simulink model "QuarkControl"  (R2018a)
settings: Solver=FixedStepAuto  StartTime=0.0  StopTime=20  FixedStep=0.004  RelTol=1e-3
InitFcn:
  | seed1 = rand()*1000000;
  | seed2 = rand()*1000000;
  | seed3 = rand()*1000000;
libraries: quarc_library x1
settings Model: SimulationMode=external  ExtModeTrigDuration=5000  Creator=RSamra  LastModifiedBy=李玉玲
settings SolverCC: PositivePriorityOrder=on  AutoInsertRateTranBlk=on
settings DataIOCC: LimitDataPoints=on  SaveFormat=Array  SignalLoggingSaveFormat=ModelDataLogs  ReturnWorkspaceOutputs=on
settings OptimizationCC: ExpressionDepthLimit=2147483647  InitFltsAndDblsToZero=on  LifeSpan=inf
settings DebuggingCC: UnderspecifiedInitializationDetection=Classic  MergeDetectMultiDrivingBlocksExec=none  SolverPrmCheckMsg=warning  FcnCallInpInsideContextMsg=warning  StateNameClashWarn=warning  SFUnexpectedBacktrackingDiag=warning  SFNoUnconditionalDefaultTransitionDiag=warning  SFExecutionAtInitializationDiag=none
settings HardwareCC: ProdBitPerPointer=32  ProdBitPerSizeT=32  ProdBitPerPtrDiffT=32  ProdLargestAtomicFloat=None  ProdIntDivRoundTo=Undefined  ProdEndianess=Unspecified  ProdWordSize=32  ProdHWDeviceType=32-bit Generic
settings ModelReferenceCC: PropagateSignalLabelsOutOfModel=off
settings SFSimCC: SimParseCustomCode=off
settings RTWCC: SystemTargetFile=quarc_win64.tlc  TemplateMakefile=quarc_default_tmf  Description=QUARC Win64 Target
settings CodeAppCC: StateflowObjectComments=on
settings STFCustomTargetCC: TargetPreCompLibLocation=C:\PROGRA~3\QUARC\lib\2018a\win64\release  ConcurrentExecutionCompliant=on  CombineOutputUpdateFcns=on  CPPClassGenCompliant=on  GRTInterface=off  SystemTargetFile=quarc_win64.tlc
settings GRTTargetCC: TargetPreCompLibLocation=C:\PROGRA~3\QUARC\lib\2018a\win64\release  TargetLangStandard=C89/C90 (ANSI)  ParMdlRefBuildCompliant=off  CompOptLevelCompliant=off  MatFileLogging=off  UseToolchainInfoCompliant=off  ExtMode=on  ExtModeMexFile=quarc_comm
settings ConfigComp: CovMetricSettings=dw  CovSaveCumulativeToWorkspaceVar=on  CovSaveSingleToWorkspaceVar=on  CovExternalEMLEnable=off

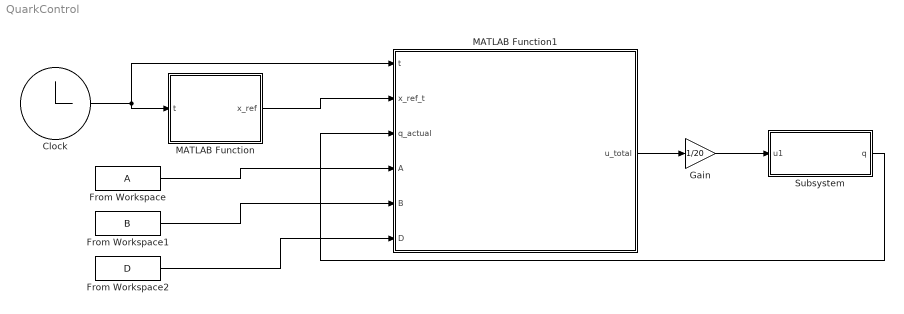
== system QuarkControl ==
  Clock : Clock
      settings: Decimation=99999999
  From Workspace : FromWorkspace  VariableName=A  SampleTime=0
  From Workspace1 : FromWorkspace  VariableName=B  SampleTime=0
  From Workspace2 : FromWorkspace  VariableName=D  SampleTime=0
  Gain : Gain  Gain=1/20
  MATLAB Function : MATLAB Function  TreatAsAtomicUnit=on
  MATLAB Function1 : MATLAB Function  TreatAsAtomicUnit=on
  Subsystem : Subsystem
  wires:
  Clock/1 -> MATLAB Function1/1(t), MATLAB Function/1(t)
  MATLAB Function/1(x_ref) -> MATLAB Function1/2(x_ref_t)
  MATLAB Function1/1(u_total) -> Gain/1
  Subsystem/1(q) -> MATLAB Function1/3(q_actual)
  From Workspace/1 -> MATLAB Function1/4(A)
  From Workspace1/1 -> MATLAB Function1/5(B)
  From Workspace2/1 -> MATLAB Function1/6(D)
  Gain/1 -> Subsystem/1(u1)

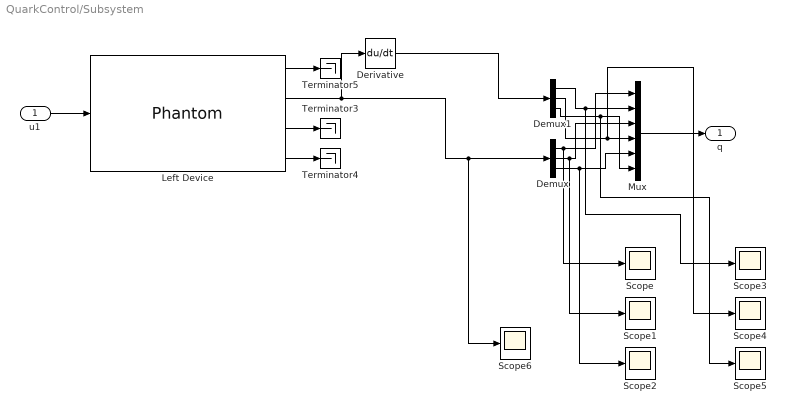
== system QuarkControl/Subsystem ==
  u1 : Inport  PortDimensions=[3 1]
  Demux : Demux  Outputs=3
  Demux1 : Demux  Outputs=3
  Derivative : Derivative
  Left Device : quarc_library/Devices/Third-Party/SensAble/Phantom/Phantom  device_name=Default Device  output_type=Joint and Gimbal Angles  input_type=Joint space  velocity_limit_option=off  velocity_limit=1200  is_7dof=off  sample_time=0.004
      settings: AttributesFormatString=(%<device_name>)  SourceProductName=QUARC Targets
  Mux : Mux  Inputs=6
  Scope{,1..6} (7 alike) : Scope
  Terminator3 : Terminator
  Terminator4 : Terminator
  Terminator5 : Terminator
  q : Outport  PortDimensions=[6 1]
  wires:
  u1/1 -> Left Device/1
  Left Device/2 -> Scope6/1, Demux/1, Derivative/1
  Derivative/1 -> Demux1/1
  Left Device/3 -> Terminator3/1
  Left Device/4 -> Terminator4/1
  Left Device/1 -> Terminator5/1
  Demux/1 -> Scope/1, Mux/1
  Demux/2 -> Scope1/1, Mux/3
  Demux/3 -> Scope2/1, Mux/5
  Demux1/1 -> Scope3/1, Mux/2
  Demux1/2 -> Scope4/1, Mux/4
  Demux1/3 -> Scope5/1, Mux/6
  Mux/1 -> q/1

== matlab function QuarkControl/MATLAB Function1 ==
  data: t input; u_total output; x_ref_t input; q_actual input; A input; B input; D input
function u_total = koopman_lqr_controller(t, x_ref_t, q_actual, A, B, D)
% 描述:
% Koopman LQR 轨迹跟踪控制器 (前馈 + 反馈)
%
% 输入:
%   t:        当前时间 (来自 Clock)
%   x_ref_t:  当前时刻的期望轨迹 [6x1] (来自模块1)
%   q_actual: 当前时刻的实际状态 [6x1] (来自系统反馈)
%   A:        Koopman 状态矩阵 [z_dim x z_dim] (来自工作区)
%   B:        Koopman 控制矩阵 [z_dim x p] (来自工作区)
%   D:        特征选择矩阵 [N x P] (来自工作区)
%
% 输出:
%   u_total:  计算得到的控制力矩 [p x 1]

% --- 1. 定义系统维度 ---
n = size(q_actual, 1); % n=6
p = size(B, 2);      % p=3
N = size(D, 1);      % N
z_dim = n + N;

% --- 2. 时间检查 (按要求 t < 10 时输出 0) ---
if t < 10.0
    u_total = zeros(p, 1);
    return;
end

% --- 3. 定义控制器内部参数 (使用 persistent 提高效率) ---
% persistent 变量只在第一次运行时计算一次，
% 避免在每个Simulink步长都重新计算LQR增益。

persistent K_lqr B_pinv is_initialized;

if isempty(is_initialized)
    % 1. 定义C矩阵 (如您所要求)
    % C_model = [eye(n), zeros(n, N)]; % (C矩阵在控制器中并未使用)
    
    % 2. 定义LQR惩罚矩阵 Q 和 R
    Q = zeros(z_dim, z_dim);
    % [q1, dq1, q2, dq2, q3, dq3] 的惩罚
    Q_x_diag = [100; 0; 100; 0; 100; 0]; 
    Q(1:n, 1:n) = diag(Q_x_diag);
    
    % R 矩阵 (控制惩罚)
    % 注：R=0 在 dlqr 中是不允许的 (必须是正定)。
    % 使用一个很小的值 (1e-4) 来代替 0。
    R = 0 * eye(p);
    
    % 3. 计算 LQR 增益 (需要 Control System Toolbox)
    K_lqr = dlqr(double(A), double(B), double(Q), double(R));
    
    % 4. 计算 B 的伪逆 (用于前馈)
    B_pinv = pinv(double(B));
    
    is_initialized = true;
end

% --- 4. 仿真步长 (必须与您的Simulink求解器步长一致!) ---
dt = 0.004;

% --- 5. 计算前馈控制 (u_ff) ---
% u_ff(t) = pinv(B) * (z_ref(t+1) - A * z_ref(t))

% 5.1. 抬升当前期望状态 z_ref(t)
z_ref_t = lift_state(x_ref_t, D, n);

% 5.2. 计算下一时刻的期望状态 x_ref(t+1)
t_next = t + dt;
x_ref_t_next = generate_reference_internal(t_next, n);

% 5.3. 抬升下一时刻的期望状态 z_ref(t+1)
z_ref_t_next = lift_state(x_ref_t_next, D, n);

% 5.4. 计算前馈控制
u_ff = B_pinv * (z_ref_t_next - A * z_ref_t);

% --- 6. 计算反馈控制 (u_fb) ---
% u_fb(t) = -K_lqr * (z_actual(t) - z_ref(t))

% 6.1. 抬升当前实际状态 z_actual(t)
z_actual = lift_state(q_actual, D, n);

% 6.2. 计算状态误差
z_error = z_actual - z_ref_t;

% 6.3. 计算反馈控制
u_fb = -K_lqr * z_error;

% --- 7. 计算总控制 ---
u_total = u_ff + u_fb;

end

% =========================================================================
% --- 内部辅助函数 (Internal Helper Functions) ---
% =========================================================================

function z = lift_state(x, D_in, n_in)
    % 辅助函数：将 [n x 1] 的状态 x 抬升到 [z_dim x 1] 的 z
    
    % lift_function 需要 (m x n) 输入, 即 (1 x 6)
    phi_x_row = lift_function(x'); 
    
    % 转换为 (P x 1)
    phi_x_col = phi_x_row';
    
    % z = [x; D*Phi]
    z = [x(1:n_in, 1); D_in * phi_x_col];
end


function x_ref_internal = generate_reference_internal(t_in, n_in)
    % 辅助函数：计算 t_in 时刻的期望轨迹
    % (与模块1的逻辑完全相同)
    
    % --- 1. 定义轨迹参数 ---
    f_pos = 0.1;   % 频率 (Hz)
    omega = 2 * pi * f_pos; % 角频率 (rad/s)
    A1 = 0.3; B1 = 0.0;   % 关节 1
    A2 = 0.2; B2 = 0.865; % 关节 2
    A3 = 0.1; B3 = 1.045; % 关节 3

    % --- 2. 计算位置和速度 ---
    x_ref_internal = zeros(n_in, 1); % 列向量

    pos_ref_1 = A1 * sin(omega * t_in) + B1;
    vel_ref_1 = A1 * omega * cos(omega * t_in);
    pos_ref_2 = A2 * sin(omega * t_in) + B2;
    vel_ref_2 = A2 * omega * cos(omega * t_in);
    pos_ref_3 = A3 * sin(omega * t_in) + B3;
    vel_ref_3 = A3 * omega * cos(omega * t_in);

    % --- 3. 构造输出向量 ---
    x_ref_internal(1) = pos_ref_1;
    x_ref_internal(2) = vel_ref_1;
    x_ref_internal(3) = pos_ref_2;
    x_ref_internal(4) = vel_ref_2;
    x_ref_internal(5) = pos_ref_3;
    x_ref_internal(6) = vel_ref_3;
end


% =========================================================================
% --- 【嵌入的完整基函数库 (已修正)】 ---
% =========================================================================

function y = lift_function(q)
% LIFT_FUNCTION - 635 维扩充版 (a1 - a21)
% 【嵌入版本：用于MATLAB Function模块】

% --- 1. 提取状态 ---
q1=q(:,1);  dq1=q(:,2);
q2=q(:,3);  dq2=q(:,4);
q3=q(:,5);  dq3=q(:,6);

% --- 2. 基础项 (a1) ---
a1 = [q1, dq1, q2, dq2, q3, dq3, ones(size(q1,1),1)];

% --- 3. 三角函数辅助变量 (a2, a3) ---
c1=cos(q1); s1=sin(q1);
c2=cos(q2); s2=sin(q2);
c3=cos(q3); s3=sin(q3);
c2p3 = cos(q2+q3);
s2p3 = sin(q2+q3);
c2m3 = cos(q2-q3);
s2m3 = sin(q2-q3);

a2 = [s1, c1, s2, c2, s3, c3, c2p3, s2p3, c2m3, s2m3, ...
      c2.*s2, c3.*s3, c2p3.*s2p3, s2.*s3, c2.*c3, s2.*s2p3];

c2q2 = cos(2*q2);  s2q2 = sin(2*q2);
c2q3 = cos(2*q3);  s2q3 = sin(2*q3);
c3q2 = cos(3*q2);  s3q2 = sin(3*q2);
c3q3 = cos(3*q3);  s3q3 = sin(3*q3);
c2q2p3 = cos(2*q2+q3);  s2q2p3 = sin(2*q2+q3);
c2q2m3 = cos(2*q2-q3);  s2q2m3 = sin(2*q2-q3);
cq2p2q3 = cos(q2+2*q3);  sq2p2q3 = sin(q2+2*q3);
c2q2p2q3 = cos(2*q2+2*q3); s2q2p2q3 = sin(2*q2+2*q3);

a3 = [c2q2, s2q2, c2q3, s2q3, c3q2, s3q2, c3q3, s3q3, ...
      c2q2p3, s2q2p3, c2q2m3, s2q2m3, cq2p2q3, sq2p2q3, ...
      c2q2p2q3, s2q2p2q3, ...
      cos(q1+q2), sin(q1+q2), cos(q1+q3), sin(q1+q3), ...
      cos(q1+q2+q3), sin(q1+q2+q3), cos(2*(q2+q3)), sin(2*(q2+q3))];

% --- 4. 特征组 a4 - a18 ---
a4 = [c2.^2, c3.^2, c2p3.^2, c2m3.^2, ...
      c2.*c3, c2.*c2p3, c3.*c2p3, c2.*c2m3, ...
      s2.^2, s3.^2, s2p3.^2, s2m3.^2, ...
      s2.*s3, s2.*s2p3, c2q2.*c2q3, ...
      (c2.^2).*(c2p3.^2), c2.^3, c2p3.^3, c3.^3, ...
      c2.*c3.^2, c2p3.*c3.^2, c3.^4];

a5 = [s2q2, s2q2p3, sin(2*q2+2*q3), s2q2m3, sin(2*(q2-q3)), ...
      c2.*s2, c3.*s3, c2p3.*s2p3, c2m3.*s2m3, ...
      c2.*s2p3, s2.*c2p3, c2.*s3, s3.*c2p3, ...
      c2.^2.*c2p3, c2.*c2p3.^2, c2.^2.*c3, c3.^2.*c2p3, ...
      c2.*c3.*c2p3, s2.*s3.*s2p3, ...
      c2q2.*c3, c2.*c2q3, s2q2.*s3, s3.*c2q3, s2q3.*c2, ...
      sin(q2).*cos(q2).*cos(q3), sin(q3).*cos(q2+q3)];

a6 = [dq1.*c2, dq1.*s2, dq1.*c3, dq1.*s3, ...
      dq1.*c2p3, dq1.*s2p3, dq1.*c2m3, dq1.*s2m3, ...
      dq1.*c2.^2, dq1.*c2p3.^2, dq1.*c2.*c2p3, dq1.*c2.*c3, ...
      dq1.*c2.*s2, dq1.*s2q2, dq1.*s2q2p3, dq1.*s3, ...
      dq1.*c2q2, dq1.*c2q3, dq1.*s2q3, dq1.*c3.*s3, ...
      dq1.^2.*c2, dq1.^2.*c2p3, dq1.^2.*s2, dq1.^2.*c3, ...
      dq1.*c3.^2, dq1.*s3.^2, dq1.*c2q3];

a7 = [dq1.*s2, dq2.*s2, dq3.*s2, dq1.*s3, dq2.*s3, dq3.*s3, ...
      dq1.*s2p3, dq2.*s2p3, dq3.*s2p3, dq1.*s2m3, dq2.*s2m3, dq3.*s2m3, ...
      dq1.*c2, dq2.*c2, dq3.*c2, dq1.*c3, dq2.*c3, dq3.*c3, ...
      dq2.*s2q2, dq3.*s2q3, dq2.*c2q2, dq3.*c2q3, ...
      dq1.*s2q2p3, dq2.*s2q2p3, dq3.*s2q3, dq3.*c3q3, ...
      dq2.^2.*s2, dq3.^2.*s3, dq2.^2.*c2, dq3.^2.*c3, ...
      dq1.*dq2.*s2, dq2.*dq3.*s3, dq3.*s3.^2, dq3.*c3.^2, ...
      dq2.*c2.*c3, dq3.*s2.*s3];

a8 = [dq1.*dq2, dq1.*dq3, dq2.*dq3, ...
      s3.*dq1.*dq2, s3.*dq2.*dq3, s3.*dq1.*dq3, ...
      s2.*dq1.*dq2, s2.*dq2.*dq3, s2.*dq1.*dq3, ...
      s2q2.*dq1.*dq2, s2q2.*dq2.*dq3, s2q3.*dq2.*dq3, ...
      c2.*dq1.*dq2, c3.*dq2.*dq3, c2p3.*dq1.*dq3, ...
      dq1.*dq2.*dq3, dq1.*dq2.*s2p3, dq2.*dq3.*c3, ...
      (dq1.*dq2).*c2.^2, (dq2.*dq3).*c3.^2, ...
      (dq1.*dq3).*c2p3, dq1.*dq2.*c2.*c3, ...
      dq2.*dq3.*s2.*s3, (dq1.*dq2.*dq3).*s3, ...
      c3.*dq1.*dq3, s3.*dq1.*dq3.^2, dq2.*dq3.*c3.^2, ...
      dq2.*dq3.*s3.^2, c2q3.*dq2.*dq3];

a9 = [dq1.^2, dq2.^2, dq3.^2, ...
      dq1.^2.*c2, dq1.^2.*s2, dq2.^2.*c3, dq2.^2.*s3, dq3.^2.*c3, dq3.^2.*s3, ...
      s3.*dq3.^2, s3.*dq2.^2, s2.*dq1.^2, ...
      dq1.^3, dq2.^3, dq3.^3, ...
      dq1.^2.*dq2, dq1.^2.*dq3, dq2.^2.*dq3, ...
      sqrt(abs(dq2)), sqrt(abs(dq3)), ...
      sign(dq2).*dq2.^2, sign(dq3).*dq3.^2, ...
      dq2.^2.*c2.^2, dq3.^2.*c3.^2, ...
      dq3.^2.*s3.^2, dq3.^2.*c2q3, dq3.^3.*s3, dq3.^3.*c3, ...
      abs(dq3).^1.5, dq3.^2.*sign(dq3)];

a10 = [q1.^2, q2.^2, q3.^2, q1.*q2, q1.*q3, q2.*q3, ...
       q1.*dq1, q2.*dq2, q3.*dq3, q1.*dq2, q1.*dq3, q2.*dq1, ...
       q2.^3, q3.^3, q2.*q3.^2, q3.^4, ...
       q2.^2.*dq2, q3.^2.*dq3, (q2+q3).*dq2, q3.*dq2, ...
       q3.^2.*dq2, q3.^3.*dq3];

a11 = [c2, c2p3, c3, c2+c2p3, c2-c2p3, ...
       q2.*c2, q3.*c2p3, q3.*c3, ...
       dq2.*c2, dq3.*c2p3, c2.*c2p3, s2.*s2p3, ...
       dq2.*s2, dq3.*s3, (c2+c2p3).^2, ...
       q3.*s3, q3.^2.*c3, dq3.*c3, dq3.*s2p3, ...
       c3.*(c2+c2p3), s3.*(s2+s2p3)];

sd1 = sign(dq1); sd2 = sign(dq2); sd3 = sign(dq3);
a12 = [sd1.*dq1, sd2.*dq2, sd3.*dq3, ...
       sd1.*abs(dq1), sd2.*abs(dq2), sd3.*abs(dq3), ...
       dq1.*abs(dq1), dq2.*abs(dq2), dq3.*abs(dq3), ...
       tanh(10*dq1), tanh(10*dq2), tanh(10*dq3), ...
       dq1./(1+abs(dq1)), dq2./(1+abs(dq2)), dq3./(1+abs(dq3)), ...
       zeros(size(dq2)), zeros(size(dq3)), zeros(size(dq2)), zeros(size(dq3)), ... % 占位符 for max/min
       tanh(5*dq3), tanh(20*dq3), sd3.*abs(dq3).^1.5];

a13 = [dq1.*c2.^2, dq1.*c2p3.^2, dq1.*c2.*c2p3, dq1.*c3.^2, ...
       dq2.*c3, dq2.*c3.^2, dq3.*c3, dq3.*c3.^2, ...
       dq2.*(c2+c2p3), dq3.*(c2+c2p3), ...
       sd1.*dq1.*c2, sd2.*dq2.*c3, sd3.*dq3.*c3, ...
       dq1.*dq2.*c2, dq2.*dq3.*c3, ...
       abs(dq2).*c2, abs(dq3).*c3, dq2.*abs(dq2).*s2, ...
       dq3.*c3.^3, dq3.*s3.^2, abs(dq3).*s3, ...
       dq3.*(c2+c2p3), sd3.*dq3.*s3];

h_denom1 = 1./(1 + 0.1*c2.^2 + 0.1*c2p3.^2);
h_denom2 = 1./(1 + 0.1*c3.^2);
h_denom3 = 1./(1 + 0.05*c3.^2 + 0.05*c2p3.^2);

a14 = [h_denom1, h_denom2, h_denom3, ...
       h_denom1.*dq1, h_denom2.*dq2, h_denom2.*dq3, h_denom3.*dq3, ...
       h_denom1.*c2, h_denom1.*c2p3, h_denom2.*c3, ...
       h_denom1.^2, h_denom2.^2, h_denom3.^2, ...
       h_denom1.*c2.^2, h_denom2.*c3.^2, h_denom3.*c3, ...
       h_denom1.*dq1.^2, h_denom2.*dq2.^2, h_denom1.*dq2, ...
       h_denom2.*dq3.^2, h_denom3.*dq2.*dq3];

a15 = [q2.*dq2.^2, q3.*dq3.^2, q2.*dq3.^2, ...
       dq1.^2.*dq2, dq1.^2.*dq3, dq2.*dq3.^2, dq1.*dq2.^2, ...
       q2.*c2.*dq2, q3.*c3.*dq3, q2.*s2.*dq2, ...
       c2.*dq1.*dq2, c3.*dq2.*dq3, s2.*dq1.^2, ...
       dq1.*dq2.*s2p3, dq1.*dq3.*c2p3, ...
       q2.*dq2.*c2, q3.*dq3.*c3, dq2.^2.*s2q2, ...
       q3.*dq3.^2.*c3, q3.*dq3.^2.*s3, q3.^2.*dq3.*c3, ...
       dq3.^2.*c3, dq1.*dq3.^2];

% 【已修正】dq3./(1DEN+abs(c3)) -> dq3./(1+abs(c3))
a16 = [zeros(size(dq2)), zeros(size(dq3)), ... % 占位符 for max/min
       dq2.*(1+c2.^2), dq3.*(1+c3.^2), ...
       dq2.*(1+0.5*c2p3.^2), dq3.*(1+0.5*c3.^2), ...
       dq1./(1+0.1*abs(dq1)), dq2./(1+0.1*abs(dq2)), dq3./(1+0.1*abs(dq3)), ...
       dq2.*(c2+0.5*c2p3), dq3.*(c3+0.5*c2p3), ...
       dq2.*exp(-0.1*q2.^2), dq3.*exp(-0.1*q3.^2), ...
       dq1.*dq2./(1+abs(dq2)), dq2.*dq3./(1+abs(dq3)), ...
       dq2./(1+abs(sin(q3))), dq3./(1+abs(sin(q3))), ...
       dq1.*c2./(1+abs(c2)), dq2.*c3./(1+abs(c3)), ...
       (dq2+dq3).*c2p3, ...
       dq3./(1+abs(c3)), dq3.*(1+s3.^2), zeros(size(dq3)), ... % 占位符 for max/min
       dq3.*(1+abs(q3)), dq3.*exp(-0.05*abs(q3)), ...
       dq3./(1+0.2*abs(dq3)), dq3.*(c3+c2p3)];

a17 = [dq2 + 0.1*dq3, dq3 + 0.1*dq2, ...
       dq1.*(dq2+dq3), (dq1+dq2).*dq3, ...
       dq2 - 0.1*dq2.^3, dq3 - 0.1*dq3.^3, ...
       dq2.*cos(0.5*q2), dq3.*cos(0.5*q3), ...
       (dq2.*dq3)./(1+abs(dq2)+abs(dq3)), ...
       dq2.*(1-0.1*abs(dq2)), dq3.*(1-0.1*abs(dq3)), ...
       dq1+dq2+dq3, ...
       dq3 + 0.2*dq2, dq3.*(1+0.1*dq2), ...
       dq3.*sin(0.5*q3), dq3 - 0.05*dq3.^3, ...
       (dq3+dq2)./(1+abs(dq3)), dq3./(1+abs(dq2)+abs(dq3))];

a18 = [c3.*s3.*dq3, c3.^2.*s3.*dq3, s3.^2.*dq3, ...
       c2q3.*dq3, s2q3.*dq3.^2, c3q3.*dq3, ...
       dq3.*c3./(1+s3.^2), dq3.*s3./(1+c3.^2), ...
       dq2.*dq3.*c3.*s3, dq1.*dq3.*c3, ...
       q3.*c3.*s3, q3.^2.*dq3.*s3, ...
       dq3.^2.*c3.*s3, (dq2.*dq3).*c3, ...
       abs(dq3).*c3.*s3, dq3.*(c3-s3), ...
       dq3.*(c3+s3).^2, c2p3.*s2p3.*dq3, ...
       dq3.*c3.^2.*s3, q3.*dq3.*(c3+s3)];
   
% --- a19: 耦合项 (30 terms) ---
trig_basis_c = [s3, s2q2, s2q2p2q3, s2q2p3, c2.*s2p3];
vel_basis_c = [dq1.^2, dq2.^2, dq3.^2, dq1.*dq2, dq1.*dq3, dq2.*dq3];

a19_list = [];
for i = 1:size(trig_basis_c, 2)
    for j = 1:size(vel_basis_c, 2)
        a19_list = [a19_list, trig_basis_c(:, i) .* vel_basis_c(:, j)];
    end
end
a19 = a19_list;

% --- a20: 高阶多项式 (100 terms) ---
a20_g1 = [q2.^4, q3.^4, dq1.^4, dq2.^4, dq3.^4]; % 5
a20_g2 = [q2.^5, q3.^5, dq1.^5, dq2.^5, dq3.^5]; % 5
a20_g3 = [q2.^3.*dq1, q2.^3.*dq2, q2.^3.*dq3, q3.^3.*dq1, q3.^3.*dq2, q3.^3.*dq3]; % 6
a20_g4 = [q2.*dq1.^3, q2.*dq2.^3, q2.*dq3.^3, q3.*dq1.^3, q3.*dq2.^3, q3.*dq3.^3]; % 6
a20_g5 = [q2.^2.*dq1.^2, q2.^2.*dq2.^2, q2.^2.*dq3.^2, q3.^2.*dq1.^2, q3.^2.*dq2.^2, q3.^2.*dq3.^2]; % 6
a20_g6 = [dq1.^3.*dq2, dq1.^3.*dq3, dq2.^3.*dq1, dq2.^3.*dq3, dq3.^3.*dq1, dq3.^3.*dq2, ...
          dq1.^2.*dq2.^2, dq1.^2.*dq3.^2, dq2.^2.*dq3.^2, dq1.*dq2.*dq3.^2]; % 10
a20_g7 = [dq1.^4.*dq2, dq1.^4.*dq3, dq2.^4.*dq1, dq2.^4.*dq3, dq3.^4.*dq1, dq3.^4.*dq2, ...
          dq1.^3.*dq2.^2, dq1.^2.*dq2.^3, dq1.^3.*dq3.^2, dq1.^2.*dq3.^3, dq2.^3.*dq3.^2, dq2.^2.*dq3.^3]; % 12
a20_g8 = [q2.^4, q3.^4, q2.^3.*q3, q2.^2.*q3.^2, q2.*q3.^3]; % 5
a20_g9 = [q2.^5, q3.^5, q2.^4.*q3, q2.^3.*q3.^2, q2.^2.*q3.^3, q2.*q3.^4]; % 6

trig_basis_simple = [s2, c2, s3, c3, s2p3, c2p3];
vel_basis_3 = [dq1.^3, dq2.^3, dq3.^3];
a20_g10_list = [];
for i = 1:size(trig_basis_simple, 2)
    for j = 1:size(vel_basis_3, 2)
        a20_g10_list = [a20_g10_list, trig_basis_simple(:, i) .* vel_basis_3(:, j)];
    end
end
a20_g10 = a20_g10_list; % 18

trig_basis_simple_sq = [s2.^2, c2.^2, s3.^2, c3.^2, s2p3.^2, c2p3.^2];
vel_basis_2 = [dq1.^2, dq2.^2, dq3.^2];
a20_g11_list = [];
for i = 1:size(trig_basis_simple_sq, 2)
    for j = 1:size(vel_basis_2, 2)
        a20_g11_list = [a20_g11_list, trig_basis_simple_sq(:, i) .* vel_basis_2(:, j)];
    end
end
a20_g11 = a20_g11_list; % 18

a20 = [a20_g1, a20_g2, a20_g3, a20_g4, a20_g5, a20_g6, a20_g7, a20_g8, a20_g9, a20_g10, a20_g11]; % 100 terms

% --- a21: 物理交叉项 (90 terms) ---
g_basis = [c2, c2p3];
h_basis = [c2.^2, c2p3.^2, c2.*c2p3, c3, c2.*c3, c2p3.*c3];
vel_basis_3b = [dq1.^3, dq2.^3, dq3.^3, dq1.^2.*dq2, dq1.*dq2.^2, dq1.^2.*dq3, dq1.^dq3.^2, dq2.^2.*dq3, dq2.*dq3.^2];
trig_basis_simple_b = [s2, s3, s2p3];

a21_list = [];
% G * vel_poly (12 terms)
for i = 1:size(g_basis, 2)
    for j = 1:size(vel_basis_c, 2)
        a21_list = [a21_list, g_basis(:, i) .* vel_basis_c(:, j)];
    end
end
% H * vel_poly (36 terms)
for i = 1:size(h_basis, 2)
    for j = 1:size(vel_basis_c, 2)
        a21_list = [a21_list, h_basis(:, i) .* vel_basis_c(:, j)];
    end
end
% G * vel_poly_cubic (18 terms)
for i = 1:size(g_basis, 2)
    for j = 1:size(vel_basis_3b, 2)
        a21_list = [a21_list, g_basis(:, i) .* vel_basis_3b(:, j)];
    end
end
% H * vel_poly_cubic (9 terms)
for i = 1:3
    for j = 1:3
        a21_list = [a21_list, h_basis(:, i) .* vel_basis_3b(:, j)];
    end
end
% H * G ( 12 terms )
for i = 1:size(g_basis, 2)
    for j = 1:size(h_basis, 2)
        a21_list = [a21_list, g_basis(:, i) .* h_basis(:, j)];
    end
end
% H * simple_trig (18 terms)
for i = 1:size(h_basis, 2)
    for j = 1:size(trig_basis_simple_b, 2)
        a21_list = [a21_list, h_basis(:, i) .* trig_basis_simple_b(:, j)];
    end
end
% (Total 105 terms, slice to 90)
a21 = a21_list(:, 1:90);


% --- 5. 组合所有特征 ---
y = [a1, a2, a3, a4, a5, a6, a7, a8, a9, a10, a11, a12, a13, a14, a15, a16, a17, a18, a19, a20, a21];

% =========================================================================
% --- 【修正】应用 max/min 修复 (用于 Simulink/Coder) ---
% =========================================================================
% 索引基于 P=635 维计算

% 修正 a12 (max/min)
% 它们在 a12 的第 16, 17, 18, 19 位
% a1-a11 累积: 7+16+24+22+27+27+36+29+30+22+21 = 261
% 16 -> 261 + 16 = 277
% 17 -> 261 + 17 = 278
% 18 -> 261 + 18 = 279
% 19 -> 261 + 19 = 280
y(:, 277) = max(dq2, 0); 
y(:, 278) = max(dq3, 0);
y(:, 279) = min(dq2, 0);
y(:, 280) = min(dq3, 0);

% 修正 a16 (max)
% 它们在 a16 的第 1, 2, 23 位
% a1-a15 累积: 261(a1-11) + 22(a12) + 23(a13) + 21(a14) + 23(a15) = 370
% 1 -> 370 + 1 = 371
% 2 -> 370 + 2 = 372
% 23 -> 370 + 23 = 393
y(:, 371) = dq2./max(abs(c3),0.1);
y(:, 372) = dq3./max(abs(c3),0.1);
y(:, 393) = dq3./max(abs(s3),0.1);

% P=635
end

== matlab function QuarkControl/MATLAB Function ==
  data: t input; x_ref output
function x_ref = generate_reference(t)
% 描述:
% 根据时钟时间 t，生成 [6x1] 的列向量期望轨迹 x_ref。
% 
% 输入:
%   t: 当前时间 (来自Simulink Clock)
% 输出:
%   x_ref: 期望轨迹 [6x1] (q1, dq1, q2, dq2, q3, dq3)

% --- 1. 定义轨迹参数 ---
% 频率
f_pos = 0.1;   % 频率 (Hz) - 三个关节相同
omega = 2 * pi * f_pos; % 角频率 (rad/s)

% 关节 1 参数
A1 = 0.3;   % 幅值
B1 = 0.0;   % 偏置
% 关节 2 参数
A2 = 0.2;   % 幅值
B2 = 0.865; % 偏置
% 关节 3 参数
A3 = 0.1;   % 幅值
B3 = 1.045; % 偏置

% --- 2. 计算位置和速度 ---
n = 6;
x_ref = zeros(n, 1); % 确保输出是列向量

% 关节 1
pos_ref_1 = A1 * sin(omega * t) + B1;
vel_ref_1 = A1 * omega * cos(omega * t);

% 关节 2
pos_ref_2 = A2 * sin(omega * t) + B2;
vel_ref_2 = A2 * omega * cos(omega * t);

% 关节 3
pos_ref_3 = A3 * sin(omega * t) + B3;
vel_ref_3 = A3 * omega * cos(omega * t);

% --- 3. 构造输出向量 ---
x_ref(1) = pos_ref_1;
x_ref(2) = vel_ref_1;
x_ref(3) = pos_ref_2;
x_ref(4) = vel_ref_2;
x_ref(5) = pos_ref_3;
x_ref(6) = vel_ref_3;

end
